simulink library "halin"  (R2021b)
settings: Solver=VariableStepAuto  StartTime=0.0  StopTime=10.0  RelTol=1e-3
undefined symbols (not defined in the file): KHAL_CAN1ABM1E2E_flg, KHAL_CAN1EPB1E2E_flg, KHAL_CAN1EPS1E2E_flg, KHAL_CAN1ESC1E2E_flg, KHAL_CAN1ESC5E2E_flg, KHAL_CAN3BMS1E2E_flg, KHAL_CAN3BMS6E2E_flg, KHAL_CAN3CCU1E2E_flg, KHAL_CAN3CCU2E2E_flg, KHAL_CAN3MCUNF1E2E_flg, KHAL_CAN3MCUNR1E2E_flg, KHAL_CAN3Shifter1E2E_flg, KHAL_CAN3Shifter2E2E_flg, KHAL_CAN6FCM2E2E_flg, KHAL_CAN6FCM4E2E_flg, TRUE
libraries: simulink x645, FVT_lib x207, hcu_lib x59
(part 2 of 23)

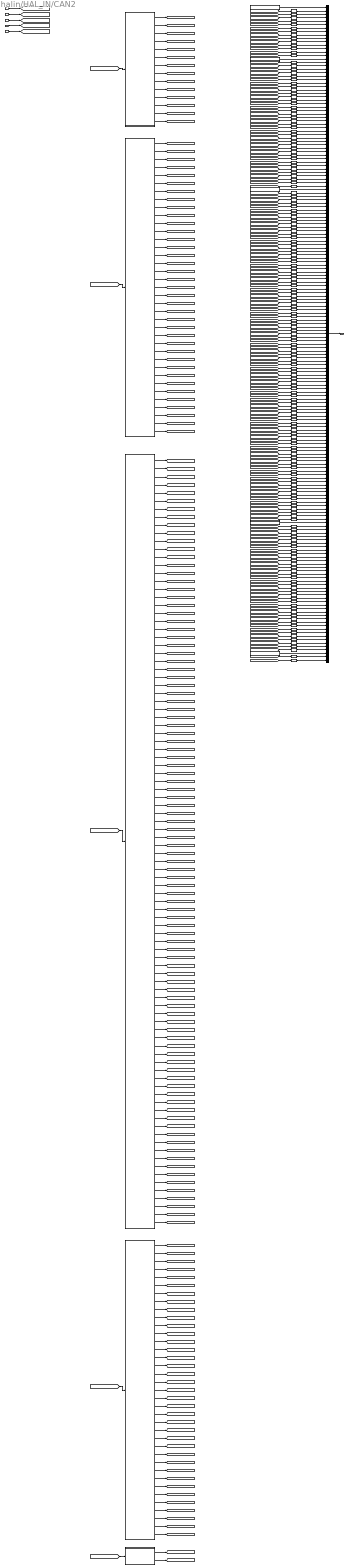
== system halin/HAL_IN/CAN2 ==
  DT_CAN2_SG_HMI1 : Inport
  DT_CAN2_SG_IVI1 : Inport  Port=2
  DT_CAN2_SG_IVI2 : Inport  Port=3
  DT_CAN2_SG_IVI3 : Inport  Port=4
  DT_CAN2_SG_METER1 : Inport  Port=5
  HMI1 : Subsystem
  IVI1 : Subsystem
  IVI2 : Subsystem
  IVI3 : Subsystem
  METER1 : Subsystem
  UnitConverter{,1..15,18..25,28..30,34,36,44..49,52..53,57,59..62,64,67,72,74..75,79..81,86,88,95,98..99,103..110,115..116,121,123..124,127..129,131,133,135..136,138,141..144,157,159,161,164,166..167,169,171,174,176,181..183} (93 alike) : DataTypeConversion  OutDataTypeStr=boolean
  UnitConverter{16..17,26..27,31..33,35,37,50,54..56,58,63,65..66,70..71,73,76..78,82..85,87,89..94,96..97,100..102,118..120,122,132,134,137,139..140,151,154..156,158,160,162..163,165,168,170,172..173,175,177,180} (64 alike) : DataTypeConversion  OutDataTypeStr=uint8
  UnitConverter{38..43,51,68,111..114,117,125..126,130,145..150,152..153,178..179,184..185} (28 alike) : DataTypeConversion  OutDataTypeStr=single
  UnitConverter69 : DataTypeConversion  OutDataTypeStr=uint32
  VHAL_CANMsgInvalidHMI1_flg : Subsystem  AncestorBlock=FVT_lib/hal/MsgTimeoutJudge_CAN_AUTOSAR
      mask help: MeasumentTrigerEvent
      mask Display: fprintf('MsgTimeoutJudge_CAN\nAUTOSAR');
  VHAL_CANMsgInvalidIVI1_flg : Subsystem  AncestorBlock=FVT_lib/hal/MsgTimeoutJudge_CAN_AUTOSAR
      mask help: MeasumentTrigerEvent
      mask Display: fprintf('MsgTimeoutJudge_CAN\nAUTOSAR');
  VHAL_CANMsgInvalidIVI2_flg : Subsystem  AncestorBlock=FVT_lib/hal/MsgTimeoutJudge_CAN_AUTOSAR
      mask help: MeasumentTrigerEvent
      mask Display: fprintf('MsgTimeoutJudge_CAN\nAUTOSAR');
  VHAL_CANMsgInvalidIVI3_flg : Subsystem  AncestorBlock=FVT_lib/hal/MsgTimeoutJudge_CAN_AUTOSAR
      mask help: MeasumentTrigerEvent
      mask Display: fprintf('MsgTimeoutJudge_CAN\nAUTOSAR');
  VHAL_CANMsgInvalidMETER1_flg : Subsystem  AncestorBlock=FVT_lib/hal/MsgTimeoutJudge_CAN_AUTOSAR
      mask help: MeasumentTrigerEvent
      mask Display: fprintf('MsgTimeoutJudge_CAN\nAUTOSAR');
  bus_creator : BusCreator  Inputs=191
  HAL_CAN2_outputs : Outport
  wires:
  DT_CAN2_SG_HMI1/1 -> [DT_CAN2_SG_HMI1]
  DT_CAN2_SG_IVI1/1 -> [DT_CAN2_SG_IVI1]
  DT_CAN2_SG_IVI2/1 -> [DT_CAN2_SG_IVI2]
  DT_CAN2_SG_IVI3/1 -> [DT_CAN2_SG_IVI3]
  DT_CAN2_SG_METER1/1 -> [DT_CAN2_SG_METER1]
  [DT_CAN2_SG_HMI1] -> HMI1/1(DT_CAN2_SG_HMI1)
  [DT_CAN2_SG_IVI1] -> IVI1/1(DT_CAN2_SG_IVI1)
  [DT_CAN2_SG_IVI2] -> IVI2/1(DT_CAN2_SG_IVI2)
  [DT_CAN2_SG_IVI3] -> IVI3/1(DT_CAN2_SG_IVI3)
  [DT_CAN2_SG_METER1] -> METER1/1(DT_CAN2_SG_METER1)
  bus_creator/1 -> HAL_CAN2_outputs/1
  VHAL_CANMsgInvalidHMI1_flg/1(Out) -> bus_creator/1
  HMI1/1(VHAL_HMIACAirIntMCmd_flg) -> [VHAL_HMIACAirIntMCmd_flg]
  UnitConverter/1 -> bus_creator/2  "VHAL_HMIACAirIntMCmd_flg"
  [VHAL_HMIACAirIntMCmd_flg] -> UnitConverter/1
  HMI1/2(VHAL_HMIACAirIntPCmd_flg) -> [VHAL_HMIACAirIntPCmd_flg]
  UnitConverter1/1 -> bus_creator/3  "VHAL_HMIACAirIntPCmd_flg"
  [VHAL_HMIACAirIntPCmd_flg] -> UnitConverter1/1
  HMI1/3(VHAL_HMIACAutoBtnCmd_flg) -> [VHAL_HMIACAutoBtnCmd_flg]
  UnitConverter2/1 -> bus_creator/4  "VHAL_HMIACAutoBtnCmd_flg"
  [VHAL_HMIACAutoBtnCmd_flg] -> UnitConverter2/1
  HMI1/4(VHAL_HMIACBtnCmd_flg) -> [VHAL_HMIACBtnCmd_flg]
  UnitConverter3/1 -> bus_creator/5  "VHAL_HMIACBtnCmd_flg"
  [VHAL_HMIACBtnCmd_flg] -> UnitConverter3/1
  HMI1/5(VHAL_HMIACFrDefogBtnCmd_flg) -> [VHAL_HMIACFrDefogBtnCmd_flg]
  UnitConverter4/1 -> bus_creator/6  "VHAL_HMIACFrDefogBtnCmd_flg"
  [VHAL_HMIACFrDefogBtnCmd_flg] -> UnitConverter4/1
  HMI1/6(VHAL_HMIACRecycleBtnCmd_flg) -> [VHAL_HMIACRecycleBtnCmd_flg]
  UnitConverter5/1 -> bus_creator/7  "VHAL_HMIACRecycleBtnCmd_flg"
  [VHAL_HMIACRecycleBtnCmd_flg] -> UnitConverter5/1
  HMI1/7(VHAL_HMIACWindDirMCmd_flg) -> [VHAL_HMIACWindDirMCmd_flg]
  UnitConverter6/1 -> bus_creator/8  "VHAL_HMIACWindDirMCmd_flg"
  [VHAL_HMIACWindDirMCmd_flg] -> UnitConverter6/1
  HMI1/8(VHAL_HMIACWindDirPCmd_flg) -> [VHAL_HMIACWindDirPCmd_flg]
  UnitConverter7/1 -> bus_creator/9  "VHAL_HMIACWindDirPCmd_flg"
  [VHAL_HMIACWindDirPCmd_flg] -> UnitConverter7/1
  HMI1/9(VHAL_HMIAutoInterLightCmd_flg) -> [VHAL_HMIAutoInterLightCmd_flg]
  UnitConverter8/1 -> bus_creator/10  "VHAL_HMIAutoInterLightCmd_flg"
  [VHAL_HMIAutoInterLightCmd_flg] -> UnitConverter8/1
  HMI1/10(VHAL_HMIBCMPostDefogBtnCmd_flg) -> [VHAL_HMIBCMPostDefogBtnCmd_flg]
  UnitConverter9/1 -> bus_creator/11  "VHAL_HMIBCMPostDefogBtnCmd_flg"
  [VHAL_HMIBCMPostDefogBtnCmd_flg] -> UnitConverter9/1
  HMI1/11(VHAL_HMIZ1SetTMCmd_flg) -> [VHAL_HMIZ1SetTMCmd_flg]
  UnitConverter10/1 -> bus_creator/12  "VHAL_HMIZ1SetTMCmd_flg"
  [VHAL_HMIZ1SetTMCmd_flg] -> UnitConverter10/1
  HMI1/12(VHAL_HMIZ1SetTPCmd_flg) -> [VHAL_HMIZ1SetTPCmd_flg]
  UnitConverter11/1 -> bus_creator/13  "VHAL_HMIZ1SetTPCmd_flg"
  [VHAL_HMIZ1SetTPCmd_flg] -> UnitConverter11/1
  HMI1/13(VHAL_HMIZ2SetTMCmd_flg) -> [VHAL_HMIZ2SetTMCmd_flg]
  UnitConverter12/1 -> bus_creator/14  "VHAL_HMIZ2SetTMCmd_flg"
  [VHAL_HMIZ2SetTMCmd_flg] -> UnitConverter12/1
  HMI1/14(VHAL_HMIZ2SetTPCmd_flg) -> [VHAL_HMIZ2SetTPCmd_flg]
  UnitConverter13/1 -> bus_creator/15  "VHAL_HMIZ2SetTPCmd_flg"
  [VHAL_HMIZ2SetTPCmd_flg] -> UnitConverter13/1
  VHAL_CANMsgInvalidIVI1_flg/1(Out) -> bus_creator/16
  IVI1/1(VHAL_AmbLighLowBatAlertSW_flg) -> [VHAL_AmbLighLowBatAlertSW_flg]
  UnitConverter14/1 -> bus_creator/17  "VHAL_AmbLighLowBatAlertSW_flg"
  [VHAL_AmbLighLowBatAlertSW_flg] -> UnitConverter14/1
  IVI1/2(VHAL_AmbLighSafetyAlertSW_flg) -> [VHAL_AmbLighSafetyAlertSW_flg]
  UnitConverter15/1 -> bus_creator/18  "VHAL_AmbLighSafetyAlertSW_flg"
  [VHAL_AmbLighSafetyAlertSW_flg] -> UnitConverter15/1
  IVI1/3(VHAL_AmbLightBrightnessSet_enum) -> [VHAL_AmbLightBrightnessSet_enum]
  UnitConverter16/1 -> bus_creator/19  "VHAL_AmbLightBrightnessSet_enum"
  [VHAL_AmbLightBrightnessSet_enum] -> UnitConverter16/1
  IVI1/4(VHAL_AmbLightColorSet_enum) -> [VHAL_AmbLightColorSet_enum]
  UnitConverter17/1 -> bus_creator/20  "VHAL_AmbLightColorSet_enum"
  [VHAL_AmbLightColorSet_enum] -> UnitConverter17/1
  IVI1/5(VHAL_AmbLightDimInDarkSW_flg) -> [VHAL_AmbLightDimInDarkSW_flg]
  UnitConverter18/1 -> bus_creator/21  "VHAL_AmbLightDimInDarkSW_flg"
  [VHAL_AmbLightDimInDarkSW_flg] -> UnitConverter18/1
  IVI1/6(VHAL_AmbLightSW_flg) -> [VHAL_AmbLightSW_flg]
  UnitConverter19/1 -> bus_creator/22  "VHAL_AmbLightSW_flg"
  [VHAL_AmbLightSW_flg] -> UnitConverter19/1
  IVI1/7(VHAL_AmbLightWlcmLightSW_flg) -> [VHAL_AmbLightWlcmLightSW_flg]
  UnitConverter20/1 -> bus_creator/23  "VHAL_AmbLightWlcmLightSW_flg"
  [VHAL_AmbLightWlcmLightSW_flg] -> UnitConverter20/1
  IVI1/8(VHAL_FCPFrEvtBtnACMaxReq_flg) -> [VHAL_FCPFrEvtBtnACMaxReq_flg]
  UnitConverter21/1 -> bus_creator/24  "VHAL_FCPFrEvtBtnACMaxReq_flg"
  [VHAL_FCPFrEvtBtnACMaxReq_flg] -> UnitConverter21/1
  IVI1/9(VHAL_FCPFrEvtBtnACReq_flg) -> [VHAL_FCPFrEvtBtnACReq_flg]
  UnitConverter22/1 -> bus_creator/25  "VHAL_FCPFrEvtBtnACReq_flg"
  [VHAL_FCPFrEvtBtnACReq_flg] -> UnitConverter22/1
  IVI1/10(VHAL_FCPFrEvtBtnAutoReq_flg) -> [VHAL_FCPFrEvtBtnAutoReq_flg]
  UnitConverter23/1 -> bus_creator/26  "VHAL_FCPFrEvtBtnAutoReq_flg"
  [VHAL_FCPFrEvtBtnAutoReq_flg] -> UnitConverter23/1
  IVI1/11(VHAL_FCPFrEvtBtnSyncReq_flg) -> [VHAL_FCPFrEvtBtnSyncReq_flg]
  UnitConverter24/1 -> bus_creator/27  "VHAL_FCPFrEvtBtnSyncReq_flg"
  [VHAL_FCPFrEvtBtnSyncReq_flg] -> UnitConverter24/1
  IVI1/12(VHAL_IVIAutoWipHSpdSWCmd_flg) -> [VHAL_IVIAutoWipHSpdSWCmd_flg]
  UnitConverter25/1 -> bus_creator/28  "VHAL_IVIAutoWipHSpdSWCmd_flg"
  [VHAL_IVIAutoWipHSpdSWCmd_flg] -> UnitConverter25/1
  IVI1/13(VHAL_IVICreateAccReqSta_enum) -> [VHAL_IVICreateAccReqSta_enum]
  UnitConverter26/1 -> bus_creator/29  "VHAL_IVICreateAccReqSta_enum"
  [VHAL_IVICreateAccReqSta_enum] -> UnitConverter26/1
  IVI1/14(VHAL_IVIDelAccReqSta_enum) -> [VHAL_IVIDelAccReqSta_enum]
  UnitConverter27/1 -> bus_creator/30  "VHAL_IVIDelAccReqSta_enum"
  [VHAL_IVIDelAccReqSta_enum] -> UnitConverter27/1
  IVI1/15(VHAL_IVIDrivingLockSWSta_flg) -> [VHAL_IVIDrivingLockSWSta_flg]
  UnitConverter28/1 -> bus_creator/31  "VHAL_IVIDrivingLockSWSta_flg"
  [VHAL_IVIDrivingLockSWSta_flg] -> UnitConverter28/1
  IVI1/16(VHAL_IVIFrTrunkUnlockReqSta_flg) -> [VHAL_IVIFrTrunkUnlockReqSta_flg]
  UnitConverter29/1 -> bus_creator/32  "VHAL_IVIFrTrunkUnlockReqSta_flg"
  [VHAL_IVIFrTrunkUnlockReqSta_flg] -> UnitConverter29/1
  IVI1/17(VHAL_IVILinkAccReqSta_flg) -> [VHAL_IVILinkAccReqSta_flg]
  UnitConverter30/1 -> bus_creator/33  "VHAL_IVILinkAccReqSta_flg"
  [VHAL_IVILinkAccReqSta_flg] -> UnitConverter30/1
  IVI1/18(VHAL_IVILinkAccSta_enum) -> [VHAL_IVILinkAccSta_enum]
  UnitConverter31/1 -> bus_creator/34  "VHAL_IVILinkAccSta_enum"
  [VHAL_IVILinkAccSta_enum] -> UnitConverter31/1
  IVI1/19(VHAL_IVILinkKeySta_enum) -> [VHAL_IVILinkKeySta_enum]
  UnitConverter32/1 -> bus_creator/35  "VHAL_IVILinkKeySta_enum"
  [VHAL_IVILinkKeySta_enum] -> UnitConverter32/1
  IVI1/20(VHAL_IVILocatedSTA_enum) -> [VHAL_IVILocatedSTA_enum]
  UnitConverter33/1 -> bus_creator/36  "VHAL_IVILocatedSTA_enum"
  [VHAL_IVILocatedSTA_enum] -> UnitConverter33/1
  IVI1/21(VHAL_IVILockSoundSWSta_flg) -> [VHAL_IVILockSoundSWSta_flg]
  UnitConverter34/1 -> bus_creator/37  "VHAL_IVILockSoundSWSta_flg"
  [VHAL_IVILockSoundSWSta_flg] -> UnitConverter34/1
  IVI1/22(VHAL_IVISWCVibModeSta_enum) -> [VHAL_IVISWCVibModeSta_enum]
  UnitConverter35/1 -> bus_creator/38  "VHAL_IVISWCVibModeSta_enum"
  [VHAL_IVISWCVibModeSta_enum] -> UnitConverter35/1
  IVI1/23(VHAL_IVIStoppingUnlockSWSta_flg) -> [VHAL_IVIStoppingUnlockSWSta_flg]
  UnitConverter36/1 -> bus_creator/39  "VHAL_IVIStoppingUnlockSWSta_flg"
  [VHAL_IVIStoppingUnlockSWSta_flg] -> UnitConverter36/1
  IVI1/24(VHAL_IVITimeCheck_enum) -> [VHAL_IVITimeCheck_enum]
  UnitConverter37/1 -> bus_creator/40  "VHAL_IVITimeCheck_enum"
  [VHAL_IVITimeCheck_enum] -> UnitConverter37/1
  IVI1/25(VHAL_IVITimeDay_DAY) -> [VHAL_IVITimeDay_DAY]
  UnitConverter38/1 -> bus_creator/41  "VHAL_IVITimeDay_DAY"
  [VHAL_IVITimeDay_DAY] -> UnitConverter38/1
  IVI1/26(VHAL_IVITimeHour_hr) -> [VHAL_IVITimeHour_hr]
  UnitConverter39/1 -> bus_creator/42  "VHAL_IVITimeHour_hr"
  [VHAL_IVITimeHour_hr] -> UnitConverter39/1
  IVI1/27(VHAL_IVITimeMinute_min) -> [VHAL_IVITimeMinute_min]
  UnitConverter40/1 -> bus_creator/43  "VHAL_IVITimeMinute_min"
  [VHAL_IVITimeMinute_min] -> UnitConverter40/1
  IVI1/28(VHAL_IVITimeMonth_MONTH) -> [VHAL_IVITimeMonth_MONTH]
  UnitConverter41/1 -> bus_creator/44  "VHAL_IVITimeMonth_MONTH"
  [VHAL_IVITimeMonth_MONTH] -> UnitConverter41/1
  IVI1/29(VHAL_IVITimeSecond_s) -> [VHAL_IVITimeSecond_s]
  UnitConverter42/1 -> bus_creator/45  "VHAL_IVITimeSecond_s"
  [VHAL_IVITimeSecond_s] -> UnitConverter42/1
  IVI1/30(VHAL_IVITimeYear_YEAR) -> [VHAL_IVITimeYear_YEAR]
  UnitConverter43/1 -> bus_creator/46  "VHAL_IVITimeYear_YEAR"
  [VHAL_IVITimeYear_YEAR] -> UnitConverter43/1
  IVI1/31(VHAL_IVIWPTCSWSta_flg) -> [VHAL_IVIWPTCSWSta_flg]
  UnitConverter44/1 -> bus_creator/47  "VHAL_IVIWPTCSWSta_flg"
  [VHAL_IVIWPTCSWSta_flg] -> UnitConverter44/1
  IVI1/32(VHAL_IVIsigScreenReqSta_flg) -> [VHAL_IVIsigScreenReqSta_flg]
  UnitConverter45/1 -> bus_creator/48  "VHAL_IVIsigScreenReqSta_flg"
  [VHAL_IVIsigScreenReqSta_flg] -> UnitConverter45/1
  IVI1/33(VHAL_LINKtoDrive_flg) -> [VHAL_LINKtoDrive_flg]
  UnitConverter46/1 -> bus_creator/49  "VHAL_LINKtoDrive_flg"
  [VHAL_LINKtoDrive_flg] -> UnitConverter46/1
  IVI1/34(VHAL_OpenDrOpenWdoSW_flg) -> [VHAL_OpenDrOpenWdoSW_flg]
  UnitConverter47/1 -> bus_creator/50  "VHAL_OpenDrOpenWdoSW_flg"
  [VHAL_OpenDrOpenWdoSW_flg] -> UnitConverter47/1
  IVI1/35(VHAL_PWCONTINUEUSE_flg) -> [VHAL_PWCONTINUEUSE_flg]
  UnitConverter48/1 -> bus_creator/51  "VHAL_PWCONTINUEUSE_flg"
  [VHAL_PWCONTINUEUSE_flg] -> UnitConverter48/1
  IVI1/36(VHAL_SmartEcoModeSW_flg) -> [VHAL_SmartEcoModeSW_flg]
  UnitConverter49/1 -> bus_creator/52  "VHAL_SmartEcoModeSW_flg"
  [VHAL_SmartEcoModeSW_flg] -> UnitConverter49/1
  IVI1/37(VHAL_UserSet_enum) -> [VHAL_UserSet_enum]
  UnitConverter50/1 -> bus_creator/53  "VHAL_UserSet_enum"
  [VHAL_UserSet_enum] -> UnitConverter50/1
  VHAL_CANMsgInvalidIVI2_flg/1(Out) -> bus_creator/54
  IVI2/1(VHAL_ACChgCurSet_A) -> [VHAL_ACChgCurSet_A]
  UnitConverter51/1 -> bus_creator/55  "VHAL_ACChgCurSet_A"
  [VHAL_ACChgCurSet_A] -> UnitConverter51/1
  IVI2/2(VHAL_AVMErrSTA_flg) -> [VHAL_AVMErrSTA_flg]
  UnitConverter52/1 -> bus_creator/56  "VHAL_AVMErrSTA_flg"
  [VHAL_AVMErrSTA_flg] -> UnitConverter52/1
  IVI2/3(VHAL_AVMOFFRecButt_flg) -> [VHAL_AVMOFFRecButt_flg]
  UnitConverter53/1 -> bus_creator/57  "VHAL_AVMOFFRecButt_flg"
  [VHAL_AVMOFFRecButt_flg] -> UnitConverter53/1
  IVI2/4(VHAL_AVMParkingmode_enum) -> [VHAL_AVMParkingmode_enum]
  UnitConverter54/1 -> bus_creator/58  "VHAL_AVMParkingmode_enum"
  [VHAL_AVMParkingmode_enum] -> UnitConverter54/1
  IVI2/5(VHAL_AVMparkingcancel_enum) -> [VHAL_AVMparkingcancel_enum]
  UnitConverter55/1 -> bus_creator/59  "VHAL_AVMparkingcancel_enum"
  [VHAL_AVMparkingcancel_enum] -> UnitConverter55/1
  IVI2/6(VHAL_AVMparkingexcute_enum) -> [VHAL_AVMparkingexcute_enum]
  UnitConverter56/1 -> bus_creator/60  "VHAL_AVMparkingexcute_enum"
  [VHAL_AVMparkingexcute_enum] -> UnitConverter56/1
  IVI2/7(VHAL_ApproachUnlockSW_flg) -> [VHAL_ApproachUnlockSW_flg]
  UnitConverter57/1 -> bus_creator/61  "VHAL_ApproachUnlockSW_flg"
  [VHAL_ApproachUnlockSW_flg] -> UnitConverter57/1
  IVI2/8(VHAL_CAASSw_enum) -> [VHAL_CAASSw_enum]
  UnitConverter58/1 -> bus_creator/62  "VHAL_CAASSw_enum"
  [VHAL_CAASSw_enum] -> UnitConverter58/1
  IVI2/9(VHAL_CDLLockButt_flg) -> [VHAL_CDLLockButt_flg]
  UnitConverter59/1 -> bus_creator/63  "VHAL_CDLLockButt_flg"
  [VHAL_CDLLockButt_flg] -> UnitConverter59/1
  IVI2/10(VHAL_CDLUnlockButt_flg) -> [VHAL_CDLUnlockButt_flg]
  UnitConverter60/1 -> bus_creator/64  "VHAL_CDLUnlockButt_flg"
  [VHAL_CDLUnlockButt_flg] -> UnitConverter60/1
  IVI2/11(VHAL_DSEATantiset_flg) -> [VHAL_DSEATantiset_flg]
  UnitConverter61/1 -> bus_creator/65  "VHAL_DSEATantiset_flg"
  [VHAL_DSEATantiset_flg] -> UnitConverter61/1
  IVI2/12(VHAL_DSEATentryfunset_flg) -> [VHAL_DSEATentryfunset_flg]
  UnitConverter62/1 -> bus_creator/66  "VHAL_DSEATentryfunset_flg"
  [VHAL_DSEATentryfunset_flg] -> UnitConverter62/1
  IVI2/13(VHAL_DSEATventreq_enum) -> [VHAL_DSEATventreq_enum]
  UnitConverter63/1 -> bus_creator/67  "VHAL_DSEATventreq_enum"
  [VHAL_DSEATventreq_enum] -> UnitConverter63/1
  IVI2/14(VHAL_Distanceunit_flg) -> [VHAL_Distanceunit_flg]
  UnitConverter64/1 -> bus_creator/68  "VHAL_Distanceunit_flg"
  [VHAL_Distanceunit_flg] -> UnitConverter64/1
  IVI2/15(VHAL_ESCSWCmd_enum) -> [VHAL_ESCSWCmd_enum]
  UnitConverter65/1 -> bus_creator/69  "VHAL_ESCSWCmd_enum"
  [VHAL_ESCSWCmd_enum] -> UnitConverter65/1
  IVI2/16(VHAL_FSOffSw_enum) -> [VHAL_FSOffSw_enum]
  UnitConverter66/1 -> bus_creator/70  "VHAL_FSOffSw_enum"
  [VHAL_FSOffSw_enum] -> UnitConverter66/1
  IVI2/17(VHAL_FollowMeSW_flg) -> [VHAL_FollowMeSW_flg]
  UnitConverter67/1 -> bus_creator/71  "VHAL_FollowMeSW_flg"
  [VHAL_FollowMeSW_flg] -> UnitConverter67/1
  IVI2/18(VHAL_GPSLAT_s) -> [VHAL_GPSLAT_s]
  UnitConverter68/1 -> bus_creator/72  "VHAL_GPSLAT_s"
  [VHAL_GPSLAT_s] -> UnitConverter68/1
  IVI2/19(VHAL_GPSLONG_enum) -> [VHAL_GPSLONG_enum]
  UnitConverter69/1 -> bus_creator/73  "VHAL_GPSLONG_enum"
  [VHAL_GPSLONG_enum] -> UnitConverter69/1
  IVI2/20(VHAL_HeadLampSW_enum) -> [VHAL_HeadLampSW_enum]
  UnitConverter70/1 -> bus_creator/74  "VHAL_HeadLampSW_enum"
  [VHAL_HeadLampSW_enum] -> UnitConverter70/1
  IVI2/21(VHAL_HoodLatchSW_enum) -> [VHAL_HoodLatchSW_enum]
  UnitConverter71/1 -> bus_creator/75  "VHAL_HoodLatchSW_enum"
  [VHAL_HoodLatchSW_enum] -> UnitConverter71/1
  IVI2/22(VHAL_IVIACCAdaptiveSta_flg) -> [VHAL_IVIACCAdaptiveSta_flg]
  UnitConverter72/1 -> bus_creator/76  "VHAL_IVIACCAdaptiveSta_flg"
  [VHAL_IVIACCAdaptiveSta_flg] -> UnitConverter72/1
  IVI2/23(VHAL_IVIAirIntZ3Cmd_enum) -> [VHAL_IVIAirIntZ3Cmd_enum]
  UnitConverter73/1 -> bus_creator/77  "VHAL_IVIAirIntZ3Cmd_enum"
  [VHAL_IVIAirIntZ3Cmd_enum] -> UnitConverter73/1
  IVI2/24(VHAL_IVIChargePortSWSta_flg) -> [VHAL_IVIChargePortSWSta_flg]
  UnitConverter74/1 -> bus_creator/78  "VHAL_IVIChargePortSWSta_flg"
  [VHAL_IVIChargePortSWSta_flg] -> UnitConverter74/1
  IVI2/25(VHAL_IVICreepSWReq_flg) -> [VHAL_IVICreepSWReq_flg]
  UnitConverter75/1 -> bus_creator/79  "VHAL_IVICreepSWReq_flg"
  [VHAL_IVICreepSWReq_flg] -> UnitConverter75/1
  IVI2/26(VHAL_IVIDSEATHeaterCmd_enum) -> [VHAL_IVIDSEATHeaterCmd_enum]
  UnitConverter76/1 -> bus_creator/80  "VHAL_IVIDSEATHeaterCmd_enum"
  [VHAL_IVIDSEATHeaterCmd_enum] -> UnitConverter76/1
  IVI2/27(VHAL_IVIDSEATFroEdgeHeightCmd_enum) -> [VHAL_IVIDSEATFroEdgeHeightCmd_enum]
  UnitConverter77/1 -> bus_creator/81  "VHAL_IVIDSEATFroEdgeHeightCmd_enum"
  [VHAL_IVIDSEATFroEdgeHeightCmd_enum] -> UnitConverter77/1
  IVI2/28(VHAL_IVIDSEATHeightCmd_enum) -> [VHAL_IVIDSEATHeightCmd_enum]
  UnitConverter78/1 -> bus_creator/82  "VHAL_IVIDSEATHeightCmd_enum"
  [VHAL_IVIDSEATHeightCmd_enum] -> UnitConverter78/1
  IVI2/29(VHAL_IVIDSEATMemory1Sta_flg) -> [VHAL_IVIDSEATMemory1Sta_flg]
  UnitConverter79/1 -> bus_creator/83  "VHAL_IVIDSEATMemory1Sta_flg"
  [VHAL_IVIDSEATMemory1Sta_flg] -> UnitConverter79/1
  IVI2/30(VHAL_IVIDSEATMemory2Sta_flg) -> [VHAL_IVIDSEATMemory2Sta_flg]
  UnitConverter80/1 -> bus_creator/84  "VHAL_IVIDSEATMemory2Sta_flg"
  [VHAL_IVIDSEATMemory2Sta_flg] -> UnitConverter80/1
  IVI2/31(VHAL_IVIDSEATMemoryOPTCLSSta_flg) -> [VHAL_IVIDSEATMemoryOPTCLSSta_flg]
  UnitConverter81/1 -> bus_creator/85  "VHAL_IVIDSEATMemoryOPTCLSSta_flg"
  [VHAL_IVIDSEATMemoryOPTCLSSta_flg] -> UnitConverter81/1
  IVI2/32(VHAL_IVIDSEATReclineCmd_enum) -> [VHAL_IVIDSEATReclineCmd_enum]
  UnitConverter82/1 -> bus_creator/86  "VHAL_IVIDSEATReclineCmd_enum"
  [VHAL_IVIDSEATReclineCmd_enum] -> UnitConverter82/1
  IVI2/33(VHAL_IVIDSEATSlideCmd_enum) -> [VHAL_IVIDSEATSlideCmd_enum]
  UnitConverter83/1 -> bus_creator/87  "VHAL_IVIDSEATSlideCmd_enum"
  [VHAL_IVIDSEATSlideCmd_enum] -> UnitConverter83/1
  IVI2/34(VHAL_IVIFGSAirIntCmd_enum) -> [VHAL_IVIFGSAirIntCmd_enum]
  UnitConverter84/1 -> bus_creator/88  "VHAL_IVIFGSAirIntCmd_enum"
  [VHAL_IVIFGSAirIntCmd_enum] -> UnitConverter84/1
  IVI2/35(VHAL_IVIFGSChCmd_enum) -> [VHAL_IVIFGSChCmd_enum]
  UnitConverter85/1 -> bus_creator/89  "VHAL_IVIFGSChCmd_enum"
  [VHAL_IVIFGSChCmd_enum] -> UnitConverter85/1
  IVI2/36(VHAL_IVIIONSWCmd_flg) -> [VHAL_IVIIONSWCmd_flg]
  UnitConverter86/1 -> bus_creator/90  "VHAL_IVIIONSWCmd_flg"
  [VHAL_IVIIONSWCmd_flg] -> UnitConverter86/1
  IVI2/37(VHAL_IVIISAOffsetSpd_enum) -> [VHAL_IVIISAOffsetSpd_enum]
  UnitConverter87/1 -> bus_creator/91  "VHAL_IVIISAOffsetSpd_enum"
  [VHAL_IVIISAOffsetSpd_enum] -> UnitConverter87/1
  IVI2/38(VHAL_IVINightModeSta_flg) -> [VHAL_IVINightModeSta_flg]
  UnitConverter88/1 -> bus_creator/92  "VHAL_IVINightModeSta_flg"
  [VHAL_IVINightModeSta_flg] -> UnitConverter88/1
  IVI2/39(VHAL_IVIPSEATHeaterCmd_enum) -> [VHAL_IVIPSEATHeaterCmd_enum]
  UnitConverter89/1 -> bus_creator/93  "VHAL_IVIPSEATHeaterCmd_enum"
  [VHAL_IVIPSEATHeaterCmd_enum] -> UnitConverter89/1
  IVI2/40(VHAL_IVIPSEATReclineCmd_enum) -> [VHAL_IVIPSEATReclineCmd_enum]
  UnitConverter90/1 -> bus_creator/94  "VHAL_IVIPSEATReclineCmd_enum"
  [VHAL_IVIPSEATReclineCmd_enum] -> UnitConverter90/1
  IVI2/41(VHAL_IVIPSEATSlideCmd_enum) -> [VHAL_IVIPSEATSlideCmd_enum]
  UnitConverter91/1 -> bus_creator/95  "VHAL_IVIPSEATSlideCmd_enum"
  [VHAL_IVIPSEATSlideCmd_enum] -> UnitConverter91/1
  IVI2/42(VHAL_IVIPTGModeSW_enum) -> [VHAL_IVIPTGModeSW_enum]
  UnitConverter92/1 -> bus_creator/96  "VHAL_IVIPTGModeSW_enum"
  [VHAL_IVIPTGModeSW_enum] -> UnitConverter92/1
  IVI2/43(VHAL_IVIPTGOpenHeight_enum) -> [VHAL_IVIPTGOpenHeight_enum]
  UnitConverter93/1 -> bus_creator/97  "VHAL_IVIPTGOpenHeight_enum"
  [VHAL_IVIPTGOpenHeight_enum] -> UnitConverter93/1
  IVI2/44(VHAL_IVIPTGStaSW_enum) -> [VHAL_IVIPTGStaSW_enum]
  UnitConverter94/1 -> bus_creator/98  "VHAL_IVIPTGStaSW_enum"
  [VHAL_IVIPTGStaSW_enum] -> UnitConverter94/1
  IVI2/45(VHAL_IVIPTGUSStaSW_flg) -> [VHAL_IVIPTGUSStaSW_flg]
  UnitConverter95/1 -> bus_creator/99  "VHAL_IVIPTGUSStaSW_flg"
  [VHAL_IVIPTGUSStaSW_flg] -> UnitConverter95/1
  IVI2/46(VHAL_IVIPWModeReq_enum) -> [VHAL_IVIPWModeReq_enum]
  UnitConverter96/1 -> bus_creator/100  "VHAL_IVIPWModeReq_enum"
  [VHAL_IVIPWModeReq_enum] -> UnitConverter96/1
  IVI2/47(VHAL_IVIPwrLockSW_enum) -> [VHAL_IVIPwrLockSW_enum]
  UnitConverter97/1 -> bus_creator/101  "VHAL_IVIPwrLockSW_enum"
  [VHAL_IVIPwrLockSW_enum] -> UnitConverter97/1
  IVI2/48(VHAL_IVIPwroffreq_flg) -> [VHAL_IVIPwroffreq_flg]
  UnitConverter98/1 -> bus_creator/102  "VHAL_IVIPwroffreq_flg"
  [VHAL_IVIPwroffreq_flg] -> UnitConverter98/1
  IVI2/49(VHAL_IVIRRDefReq_flg) -> [VHAL_IVIRRDefReq_flg]
  UnitConverter99/1 -> bus_creator/103  "VHAL_IVIRRDefReq_flg"
  [VHAL_IVIRRDefReq_flg] -> UnitConverter99/1
  IVI2/50(VHAL_IVIReqV2L_enum) -> [VHAL_IVIReqV2L_enum]
  UnitConverter100/1 -> bus_creator/104  "VHAL_IVIReqV2L_enum"
  [VHAL_IVIReqV2L_enum] -> UnitConverter100/1
  IVI2/51(VHAL_IVISWCRUndefinedSta_enum) -> [VHAL_IVISWCRUndefinedSta_enum]
  UnitConverter101/1 -> bus_creator/105  "VHAL_IVISWCRUndefinedSta_enum"
  [VHAL_IVISWCRUndefinedSta_enum] -> UnitConverter101/1
  IVI2/52(VHAL_IVIScreen_enum) -> [VHAL_IVIScreen_enum]
  UnitConverter102/1 -> bus_creator/106  "VHAL_IVIScreen_enum"
  [VHAL_IVIScreen_enum] -> UnitConverter102/1
  IVI2/53(VHAL_IVIStartChgreq_flg) -> [VHAL_IVIStartChgreq_flg]
  UnitConverter103/1 -> bus_creator/107  "VHAL_IVIStartChgreq_flg"
  [VHAL_IVIStartChgreq_flg] -> UnitConverter103/1
  IVI2/54(VHAL_IVIStatus_flg) -> [VHAL_IVIStatus_flg]
  UnitConverter104/1 -> bus_creator/108  "VHAL_IVIStatus_flg"
  [VHAL_IVIStatus_flg] -> UnitConverter104/1
  IVI2/55(VHAL_IVIStopChgreq_flg) -> [VHAL_IVIStopChgreq_flg]
  UnitConverter105/1 -> bus_creator/109  "VHAL_IVIStopChgreq_flg"
  [VHAL_IVIStopChgreq_flg] -> UnitConverter105/1
  IVI2/56(VHAL_IVITrailerCheckReqSta_flg) -> [VHAL_IVITrailerCheckReqSta_flg]
  UnitConverter106/1 -> bus_creator/110  "VHAL_IVITrailerCheckReqSta_flg"
  [VHAL_IVITrailerCheckReqSta_flg] -> UnitConverter106/1
  IVI2/57(VHAL_IVITrailerModeSWSta_flg) -> [VHAL_IVITrailerModeSWSta_flg]
  UnitConverter107/1 -> bus_creator/111  "VHAL_IVITrailerModeSWSta_flg"
  [VHAL_IVITrailerModeSWSta_flg] -> UnitConverter107/1
  IVI2/58(VHAL_IVITriggerreq_flg) -> [VHAL_IVITriggerreq_flg]
  UnitConverter108/1 -> bus_creator/112  "VHAL_IVITriggerreq_flg"
  [VHAL_IVITriggerreq_flg] -> UnitConverter108/1
  IVI2/59(VHAL_IVIUnlockChgreq_flg) -> [VHAL_IVIUnlockChgreq_flg]
  UnitConverter109/1 -> bus_creator/113  "VHAL_IVIUnlockChgreq_flg"
  [VHAL_IVIUnlockChgreq_flg] -> UnitConverter109/1
  IVI2/60(VHAL_IVIWIMAINSW_flg) -> [VHAL_IVIWIMAINSW_flg]
  UnitConverter110/1 -> bus_creator/114  "VHAL_IVIWIMAINSW_flg"
  [VHAL_IVIWIMAINSW_flg] -> UnitConverter110/1
  IVI2/61(VHAL_LDrvControlCommand_pct) -> [VHAL_LDrvControlCommand_pct]
  UnitConverter111/1 -> bus_creator/115  "VHAL_LDrvControlCommand_pct"
  [VHAL_LDrvControlCommand_pct] -> UnitConverter111/1
  IVI2/62(VHAL_LPasControlCommand_pct) -> [VHAL_LPasControlCommand_pct]
  UnitConverter112/1 -> bus_creator/116  "VHAL_LPasControlCommand_pct"
  [VHAL_LPasControlCommand_pct] -> UnitConverter112/1
  IVI2/63(VHAL_LRLDControlCommand_pct) -> [VHAL_LRLDControlCommand_pct]
  UnitConverter113/1 -> bus_creator/117  "VHAL_LRLDControlCommand_pct"
  [VHAL_LRLDControlCommand_pct] -> UnitConverter113/1
  IVI2/64(VHAL_LRRDControlCommand_pct) -> [VHAL_LRRDControlCommand_pct]
  UnitConverter114/1 -> bus_creator/118  "VHAL_LRRDControlCommand_pct"
  [VHAL_LRRDControlCommand_pct] -> UnitConverter114/1
  IVI2/65(VHAL_LightShowStartReq_flg) -> [VHAL_LightShowStartReq_flg]
  UnitConverter115/1 -> bus_creator/119  "VHAL_LightShowStartReq_flg"
  [VHAL_LightShowStartReq_flg] -> UnitConverter115/1
  IVI2/66(VHAL_LightShowStopReq_flg) -> [VHAL_LightShowStopReq_flg]
  UnitConverter116/1 -> bus_creator/120  "VHAL_LightShowStopReq_flg"
  [VHAL_LightShowStopReq_flg] -> UnitConverter116/1
  IVI2/67(VHAL_MFRDNBrightReq_pct) -> [VHAL_MFRDNBrightReq_pct]
  UnitConverter117/1 -> bus_creator/121  "VHAL_MFRDNBrightReq_pct"
  [VHAL_MFRDNBrightReq_pct] -> UnitConverter117/1
  IVI2/68(VHAL_OFFACMODE_enum) -> [VHAL_OFFACMODE_enum]
  UnitConverter118/1 -> bus_creator/122  "VHAL_OFFACMODE_enum"
  [VHAL_OFFACMODE_enum] -> UnitConverter118/1
  IVI2/69(VHAL_PSEATventreq_enum) -> [VHAL_PSEATventreq_enum]
  UnitConverter119/1 -> bus_creator/123  "VHAL_PSEATventreq_enum"
  [VHAL_PSEATventreq_enum] -> UnitConverter119/1
  IVI2/70(VHAL_PerdV2L_enum) -> [VHAL_PerdV2L_enum]
  UnitConverter120/1 -> bus_creator/124  "VHAL_PerdV2L_enum"
  [VHAL_PerdV2L_enum] -> UnitConverter120/1
  IVI2/71(VHAL_RFogLampSW_flg) -> [VHAL_RFogLampSW_flg]
  UnitConverter121/1 -> bus_creator/125  "VHAL_RFogLampSW_flg"
  [VHAL_RFogLampSW_flg] -> UnitConverter121/1
  IVI2/72(VHAL_RollModeSWCmd_enum) -> [VHAL_RollModeSWCmd_enum]
  UnitConverter122/1 -> bus_creator/126  "VHAL_RollModeSWCmd_enum"
  [VHAL_RollModeSWCmd_enum] -> UnitConverter122/1
  IVI2/73(VHAL_RoomLampMode_flg) -> [VHAL_RoomLampMode_flg]
  UnitConverter123/1 -> bus_creator/127  "VHAL_RoomLampMode_flg"
  [VHAL_RoomLampMode_flg] -> UnitConverter123/1
  IVI2/74(VHAL_SOCADJBUTT_flg) -> [VHAL_SOCADJBUTT_flg]
  UnitConverter124/1 -> bus_creator/128  "VHAL_SOCADJBUTT_flg"
  [VHAL_SOCADJBUTT_flg] -> UnitConverter124/1
  IVI2/75(VHAL_SOCLimitSet_pct) -> [VHAL_SOCLimitSet_pct]
  UnitConverter125/1 -> bus_creator/129  "VHAL_SOCLimitSet_pct"
  [VHAL_SOCLimitSet_pct] -> UnitConverter125/1
  IVI2/76(VHAL_SOCV2LLimit_pct) -> [VHAL_SOCV2LLimit_pct]
  UnitConverter126/1 -> bus_creator/130  "VHAL_SOCV2LLimit_pct"
  [VHAL_SOCV2LLimit_pct] -> UnitConverter126/1
  IVI2/77(VHAL_SchedChgStart_flg) -> [VHAL_SchedChgStart_flg]
  UnitConverter127/1 -> bus_creator/131  "VHAL_SchedChgStart_flg"
  [VHAL_SchedChgStart_flg] -> UnitConverter127/1
  IVI2/78(VHAL_SchedChgStop_flg) -> [VHAL_SchedChgStop_flg]
  UnitConverter128/1 -> bus_creator/132  "VHAL_SchedChgStop_flg"
  [VHAL_SchedChgStop_flg] -> UnitConverter128/1
  IVI2/79(VHAL_SchedChgbutt_flg) -> [VHAL_SchedChgbutt_flg]
  UnitConverter129/1 -> bus_creator/133  "VHAL_SchedChgbutt_flg"
  [VHAL_SchedChgbutt_flg] -> UnitConverter129/1
  IVI2/80(VHAL_SchedChglimit_pct) -> [VHAL_SchedChglimit_pct]
  UnitConverter130/1 -> bus_creator/134  "VHAL_SchedChglimit_pct"
  [VHAL_SchedChglimit_pct] -> UnitConverter130/1
  IVI2/81(VHAL_SchedChgwake_flg) -> [VHAL_SchedChgwake_flg]
  UnitConverter131/1 -> bus_creator/135  "VHAL_SchedChgwake_flg"
  [VHAL_SchedChgwake_flg] -> UnitConverter131/1
  IVI2/82(VHAL_SenstivityPosition_enum) -> [VHAL_SenstivityPosition_enum]
  UnitConverter132/1 -> bus_creator/136  "VHAL_SenstivityPosition_enum"
  [VHAL_SenstivityPosition_enum] -> UnitConverter132/1
  IVI2/83(VHAL_SetUnlockSingle_flg) -> [VHAL_SetUnlockSingle_flg]
  UnitConverter133/1 -> bus_creator/137  "VHAL_SetUnlockSingle_flg"
  [VHAL_SetUnlockSingle_flg] -> UnitConverter133/1
  IVI2/84(VHAL_TCSSWCmd_enum) -> [VHAL_TCSSWCmd_enum]
  UnitConverter134/1 -> bus_creator/138  "VHAL_TCSSWCmd_enum"
  [VHAL_TCSSWCmd_enum] -> UnitConverter134/1
  IVI2/85(VHAL_TPMSCaliButt_flg) -> [VHAL_TPMSCaliButt_flg]
  UnitConverter135/1 -> bus_creator/139  "VHAL_TPMSCaliButt_flg"
  [VHAL_TPMSCaliButt_flg] -> UnitConverter135/1
  IVI2/86(VHAL_TPMSResButt_flg) -> [VHAL_TPMSResButt_flg]
  UnitConverter136/1 -> bus_creator/140  "VHAL_TPMSResButt_flg"
  [VHAL_TPMSResButt_flg] -> UnitConverter136/1
  IVI2/87(VHAL_TurnSwTimeSet_enum) -> [VHAL_TurnSwTimeSet_enum]
  UnitConverter137/1 -> bus_creator/141  "VHAL_TurnSwTimeSet_enum"
  [VHAL_TurnSwTimeSet_enum] -> UnitConverter137/1
  IVI2/88(VHAL_WalkawayLockSW_flg) -> [VHAL_WalkawayLockSW_flg]
  UnitConverter138/1 -> bus_creator/142  "VHAL_WalkawayLockSW_flg"
  [VHAL_WalkawayLockSW_flg] -> UnitConverter138/1
  IVI2/89(VHAL_WlcmLightMode_enum) -> [VHAL_WlcmLightMode_enum]
  UnitConverter139/1 -> bus_creator/143  "VHAL_WlcmLightMode_enum"
  [VHAL_WlcmLightMode_enum] -> UnitConverter139/1
  IVI2/90(VHAL_sigAirIntenZon1Req_enum) -> [VHAL_sigAirIntenZon1Req_enum]
  UnitConverter140/1 -> bus_creator/144  "VHAL_sigAirIntenZon1Req_enum"
  [VHAL_sigAirIntenZon1Req_enum] -> UnitConverter140/1
  IVI2/91(VHAL_sigDfrstReq_flg) -> [VHAL_sigDfrstReq_flg]
  UnitConverter141/1 -> bus_creator/145  "VHAL_sigDfrstReq_flg"
  [VHAL_sigDfrstReq_flg] -> UnitConverter141/1
  IVI2/92(VHAL_sigFaceReq_flg) -> [VHAL_sigFaceReq_flg]
  UnitConverter142/1 -> bus_creator/146  "VHAL_sigFaceReq_flg"
  [VHAL_sigFaceReq_flg] -> UnitConverter142/1
  IVI2/93(VHAL_sigFootReq_flg) -> [VHAL_sigFootReq_flg]
  UnitConverter143/1 -> bus_creator/147  "VHAL_sigFootReq_flg"
  [VHAL_sigFootReq_flg] -> UnitConverter143/1
  IVI2/94(VHAL_sigRecircReq_flg) -> [VHAL_sigRecircReq_flg]
  UnitConverter144/1 -> bus_creator/148  "VHAL_sigRecircReq_flg"
  [VHAL_sigRecircReq_flg] -> UnitConverter144/1
  IVI2/95(VHAL_sigSetTempZon1Req_C) -> [VHAL_sigSetTempZon1Req_C]
  UnitConverter145/1 -> bus_creator/149  "VHAL_sigSetTempZon1Req_C"
  [VHAL_sigSetTempZon1Req_C] -> UnitConverter145/1
  IVI2/96(VHAL_sigSetTempZon2Req_C) -> [VHAL_sigSetTempZon2Req_C]
  UnitConverter146/1 -> bus_creator/150  "VHAL_sigSetTempZon2Req_C"
  [VHAL_sigSetTempZon2Req_C] -> UnitConverter146/1
  VHAL_CANMsgInvalidIVI3_flg/1(Out) -> bus_creator/151
  IVI3/1(VHAL_IVICLBlowerYSta_pct) -> [VHAL_IVICLBlowerYSta_pct]
  UnitConverter147/1 -> bus_creator/152  "VHAL_IVICLBlowerYSta_pct"
  [VHAL_IVICLBlowerYSta_pct] -> UnitConverter147/1
  IVI3/2(VHAL_IVICLBlowerZSta_pct) -> [VHAL_IVICLBlowerZSta_pct]
  UnitConverter148/1 -> bus_creator/153  "VHAL_IVICLBlowerZSta_pct"
  [VHAL_IVICLBlowerZSta_pct] -> UnitConverter148/1
  IVI3/3(VHAL_IVICRBlowerYSta_pct) -> [VHAL_IVICRBlowerYSta_pct]
  UnitConverter149/1 -> bus_creator/154  "VHAL_IVICRBlowerYSta_pct"
  [VHAL_IVICRBlowerYSta_pct] -> UnitConverter149/1
  IVI3/4(VHAL_IVICRBlowerZSta_pct) -> [VHAL_IVICRBlowerZSta_pct]
  UnitConverter150/1 -> bus_creator/155  "VHAL_IVICRBlowerZSta_pct"
  [VHAL_IVICRBlowerZSta_pct] -> UnitConverter150/1
  IVI3/5(VHAL_IVIDrBlowerModeSta_enum) -> [VHAL_IVIDrBlowerModeSta_enum]
  UnitConverter151/1 -> bus_creator/156  "VHAL_IVIDrBlowerModeSta_enum"
  [VHAL_IVIDrBlowerModeSta_enum] -> UnitConverter151/1
  IVI3/6(VHAL_IVIDrBlowerYSta_pct) -> [VHAL_IVIDrBlowerYSta_pct]
  UnitConverter152/1 -> bus_creator/157  "VHAL_IVIDrBlowerYSta_pct"
  [VHAL_IVIDrBlowerYSta_pct] -> UnitConverter152/1
  IVI3/7(VHAL_IVIDrBlowerZSta_pct) -> [VHAL_IVIDrBlowerZSta_pct]
  UnitConverter153/1 -> bus_creator/158  "VHAL_IVIDrBlowerZSta_pct"
  [VHAL_IVIDrBlowerZSta_pct] -> UnitConverter153/1
  IVI3/8(VHAL_IVIHMICustmiFunSta_enum) -> [VHAL_IVIHMICustmiFunSta_enum]
  UnitConverter154/1 -> bus_creator/159  "VHAL_IVIHMICustmiFunSta_enum"
  [VHAL_IVIHMICustmiFunSta_enum] -> UnitConverter154/1
  IVI3/9(VHAL_IVIHMICustmiKEYSta_enum) -> [VHAL_IVIHMICustmiKEYSta_enum]
  UnitConverter155/1 -> bus_creator/160  "VHAL_IVIHMICustmiKEYSta_enum"
  [VHAL_IVIHMICustmiKEYSta_enum] -> UnitConverter155/1
  IVI3/10(VHAL_IVILSEATventCmd_enum) -> [VHAL_IVILSEATventCmd_enum]
  UnitConverter156/1 -> bus_creator/161  "VHAL_IVILSEATventCmd_enum"
  [VHAL_IVILSEATventCmd_enum] -> UnitConverter156/1
  IVI3/11(VHAL_IVIMLFMostCmd_flg) -> [VHAL_IVIMLFMostCmd_flg]
  UnitConverter157/1 -> bus_creator/162  "VHAL_IVIMLFMostCmd_flg"
  [VHAL_IVIMLFMostCmd_flg] -> UnitConverter157/1
  IVI3/12(VHAL_IVIMLFootLiftCmd_enum) -> [VHAL_IVIMLFootLiftCmd_enum]
  UnitConverter158/1 -> bus_creator/163  "VHAL_IVIMLFootLiftCmd_enum"
  [VHAL_IVIMLFootLiftCmd_enum] -> UnitConverter158/1
  IVI3/13(VHAL_IVIMLNapModeCmd_flg) -> [VHAL_IVIMLNapModeCmd_flg]
  UnitConverter159/1 -> bus_creator/164  "VHAL_IVIMLNapModeCmd_flg"
  [VHAL_IVIMLNapModeCmd_flg] -> UnitConverter159/1
  IVI3/14(VHAL_IVIMLReclinerCmd_enum) -> [VHAL_IVIMLReclinerCmd_enum]
  UnitConverter160/1 -> bus_creator/165  "VHAL_IVIMLReclinerCmd_enum"
  [VHAL_IVIMLReclinerCmd_enum] -> UnitConverter160/1
  IVI3/15(VHAL_IVIMLRestoreCmd_flg) -> [VHAL_IVIMLRestoreCmd_flg]
  UnitConverter161/1 -> bus_creator/166  "VHAL_IVIMLRestoreCmd_flg"
  [VHAL_IVIMLRestoreCmd_flg] -> UnitConverter161/1
  IVI3/16(VHAL_IVIMLSEATventCmd_enum) -> [VHAL_IVIMLSEATventCmd_enum]
  UnitConverter162/1 -> bus_creator/167  "VHAL_IVIMLSEATventCmd_enum"
  [VHAL_IVIMLSEATventCmd_enum] -> UnitConverter162/1
  IVI3/17(VHAL_IVIMLSeatLiftCmd_enum) -> [VHAL_IVIMLSeatLiftCmd_enum]
  UnitConverter163/1 -> bus_creator/168  "VHAL_IVIMLSeatLiftCmd_enum"
  [VHAL_IVIMLSeatLiftCmd_enum] -> UnitConverter163/1
  IVI3/18(VHAL_IVIMLSldRestoreCmd_flg) -> [VHAL_IVIMLSldRestoreCmd_flg]
  UnitConverter164/1 -> bus_creator/169  "VHAL_IVIMLSldRestoreCmd_flg"
  [VHAL_IVIMLSldRestoreCmd_flg] -> UnitConverter164/1
  IVI3/19(VHAL_IVIMLSliderCmd_enum) -> [VHAL_IVIMLSliderCmd_enum]
  UnitConverter165/1 -> bus_creator/170  "VHAL_IVIMLSliderCmd_enum"
  [VHAL_IVIMLSliderCmd_enum] -> UnitConverter165/1
  IVI3/20(VHAL_IVIMLZeroGravityCmd_flg) -> [VHAL_IVIMLZeroGravityCmd_flg]
  UnitConverter166/1 -> bus_creator/171  "VHAL_IVIMLZeroGravityCmd_flg"
  [VHAL_IVIMLZeroGravityCmd_flg] -> UnitConverter166/1
  IVI3/21(VHAL_IVIMRFMostCmd_flg) -> [VHAL_IVIMRFMostCmd_flg]
  UnitConverter167/1 -> bus_creator/172  "VHAL_IVIMRFMostCmd_flg"
  [VHAL_IVIMRFMostCmd_flg] -> UnitConverter167/1
  IVI3/22(VHAL_IVIMRFootLiftCmd_enum) -> [VHAL_IVIMRFootLiftCmd_enum]
  UnitConverter168/1 -> bus_creator/173  "VHAL_IVIMRFootLiftCmd_enum"
  [VHAL_IVIMRFootLiftCmd_enum] -> UnitConverter168/1
  IVI3/23(VHAL_IVIMRNapModeCmd_flg) -> [VHAL_IVIMRNapModeCmd_flg]
  UnitConverter169/1 -> bus_creator/174  "VHAL_IVIMRNapModeCmd_flg"
  [VHAL_IVIMRNapModeCmd_flg] -> UnitConverter169/1
  IVI3/24(VHAL_IVIMRReclinerCmd_enum) -> [VHAL_IVIMRReclinerCmd_enum]
  UnitConverter170/1 -> bus_creator/175  "VHAL_IVIMRReclinerCmd_enum"
  [VHAL_IVIMRReclinerCmd_enum] -> UnitConverter170/1
  IVI3/25(VHAL_IVIMRRestoreCmd_flg) -> [VHAL_IVIMRRestoreCmd_flg]
  UnitConverter171/1 -> bus_creator/176  "VHAL_IVIMRRestoreCmd_flg"
  [VHAL_IVIMRRestoreCmd_flg] -> UnitConverter171/1
  IVI3/26(VHAL_IVIMRSEATventCmd_enum) -> [VHAL_IVIMRSEATventCmd_enum]
  UnitConverter172/1 -> bus_creator/177  "VHAL_IVIMRSEATventCmd_enum"
  [VHAL_IVIMRSEATventCmd_enum] -> UnitConverter172/1
  IVI3/27(VHAL_IVIMRSeatLiftCmd_enum) -> [VHAL_IVIMRSeatLiftCmd_enum]
  UnitConverter173/1 -> bus_creator/178  "VHAL_IVIMRSeatLiftCmd_enum"
  [VHAL_IVIMRSeatLiftCmd_enum] -> UnitConverter173/1
  IVI3/28(VHAL_IVIMRSldRestoreCmd_flg) -> [VHAL_IVIMRSldRestoreCmd_flg]
  UnitConverter174/1 -> bus_creator/179  "VHAL_IVIMRSldRestoreCmd_flg"
  [VHAL_IVIMRSldRestoreCmd_flg] -> UnitConverter174/1
  IVI3/29(VHAL_IVIMRSliderCmd_enum) -> [VHAL_IVIMRSliderCmd_enum]
  UnitConverter175/1 -> bus_creator/180  "VHAL_IVIMRSliderCmd_enum"
  [VHAL_IVIMRSliderCmd_enum] -> UnitConverter175/1
  IVI3/30(VHAL_IVIMRZeroGravityCmd_flg) -> [VHAL_IVIMRZeroGravityCmd_flg]
  UnitConverter176/1 -> bus_creator/181  "VHAL_IVIMRZeroGravityCmd_flg"
  [VHAL_IVIMRZeroGravityCmd_flg] -> UnitConverter176/1
  IVI3/31(VHAL_IVIPsBlowerModeSta_enum) -> [VHAL_IVIPsBlowerModeSta_enum]
  UnitConverter177/1 -> bus_creator/182  "VHAL_IVIPsBlowerModeSta_enum"
  [VHAL_IVIPsBlowerModeSta_enum] -> UnitConverter177/1
  IVI3/32(VHAL_IVIPsBlowerYSta_pct) -> [VHAL_IVIPsBlowerYSta_pct]
  UnitConverter178/1 -> bus_creator/183  "VHAL_IVIPsBlowerYSta_pct"
  [VHAL_IVIPsBlowerYSta_pct] -> UnitConverter178/1
  IVI3/33(VHAL_IVIPsBlowerZSta_pct) -> [VHAL_IVIPsBlowerZSta_pct]
  UnitConverter179/1 -> bus_creator/184  "VHAL_IVIPsBlowerZSta_pct"
  [VHAL_IVIPsBlowerZSta_pct] -> UnitConverter179/1
  IVI3/34(VHAL_IVIRSEATventCmd_enum) -> [VHAL_IVIRSEATventCmd_enum]
  UnitConverter180/1 -> bus_creator/185  "VHAL_IVIRSEATventCmd_enum"
  [VHAL_IVIRSEATventCmd_enum] -> UnitConverter180/1
  IVI3/35(VHAL_IVISnowModeCmd_flg) -> [VHAL_IVISnowModeCmd_flg]
  UnitConverter181/1 -> bus_creator/186  "VHAL_IVISnowModeCmd_flg"
  [VHAL_IVISnowModeCmd_flg] -> UnitConverter181/1
  IVI3/36(VHAL_IVIUserTakeOverAPSSta_flg) -> [VHAL_IVIUserTakeOverAPSSta_flg]
  UnitConverter182/1 -> bus_creator/187  "VHAL_IVIUserTakeOverAPSSta_flg"
  [VHAL_IVIUserTakeOverAPSSta_flg] -> UnitConverter182/1
  IVI3/37(VHAL_IVIZon1WindDirSWReqSta_flg) -> [VHAL_IVIZon1WindDirSWReqSta_flg]
  UnitConverter183/1 -> bus_creator/188  "VHAL_IVIZon1WindDirSWReqSta_flg"
  [VHAL_IVIZon1WindDirSWReqSta_flg] -> UnitConverter183/1
  VHAL_CANMsgInvalidMETER1_flg/1(Out) -> bus_creator/189
  METER1/1(VHAL_METERKPHCalcu_kph) -> [VHAL_METERKPHCalcu_kph]
  UnitConverter184/1 -> bus_creator/190  "VHAL_METERKPHCalcu_kph"
  [VHAL_METERKPHCalcu_kph] -> UnitConverter184/1
  METER1/2(VHAL_ODOMETER_km) -> [VHAL_ODOMETER_km]
  UnitConverter185/1 -> bus_creator/191  "VHAL_ODOMETER_km"
  [VHAL_ODOMETER_km] -> UnitConverter185/1
